simulink model "downCounter"  (R2016b)
settings: Solver=VariableStepAuto  StartTime=0.0  StopTime=10.0  RelTol=1e-3
settings Model: Creator=Radwa  LastModifiedBy=Radwa

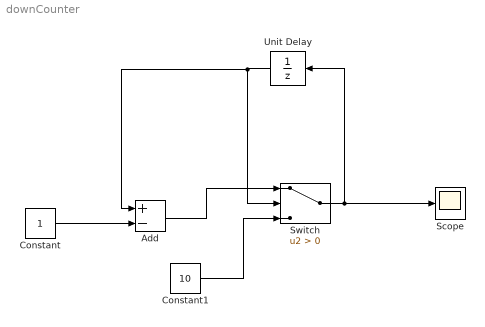
== system downCounter ==
  Add : Sum  Inputs=+-
  Constant : Constant
  Constant1 : Constant  Value=10
  Scope : Scope
  Switch : Switch  Criteria=u2 > Threshold
  Unit Delay : UnitDelay  SampleTime=-1
  wires:
  Unit Delay/1 -> Add/1, Switch/2
  Switch/1 -> Scope/1, Unit Delay/1
  Add/1 -> Switch/1
  Constant1/1 -> Switch/3
  Constant/1 -> Add/2
